simulink model "flightControlSystem"  (R2022a)
settings: Solver=ode3  StartTime=0  StopTime=TFinal  FixedStep=Ts  RelTol=1e-3  EnableMultiTasking=on
model workspace (MAT data in the model file):
  CIRCLE_PTS = [19 19 19]
  ZEROS = [0 0 0 0 0 0 0 0 0 0 0 0 ... (1444 elements, 38x38)]
undefined symbols (not defined in the file): codertarget, Controller, DiscIntNeverNeededParam, Discrete, Estimator, g, gray, init, Sensors, Time, Ts, var_acc_angle_N, var_bias_gyr_N, var_gyro_p_N, Vehicle
libraries: simulink x38, slpidlib x4, ctrlSharedLib x4, sharedtransform x3, visiontextngfix x1, parrotlib x1
(part 3 of 3)

== matlab function flightControlSystem/Image Processing System/write_or_not ==
  data: way input; way_out output; in_red input; prev_xy input; way_x output; way_y output
function [way_out, way_x, way_y] = fcn(way, in_red, prev_xy)

x = way(1);
y = way(2);
speed = way(3);

if in_red
    X = x;   Y = y;
    way_x = x;  way_y = y;
else
    X = x;  Y = y; 
    way_x = prev_xy(1);  
    way_y = prev_xy(2);
end

way_out = [X Y speed];

%fprintf('X = %f | Y = %f\n', way_x, way_y);
end

== matlab function flightControlSystem/Control System/Controller/Position Controller/Position error transformation (Earth to Body frame) ==
  data: yaw input; xy_err_earth input; xy_err_body output
function xy_err_body = fcn(yaw,xy_err_earth)

transformation = [cos(yaw), sin(yaw); -sin(yaw),  cos(yaw)];
xy_err_body = transformation * xy_err_earth;


end

== matlab function flightControlSystem/Image Processing System/speed_calculator ==
  data: way input; X output; Y output
function [X,Y] = fcn(way)

x = way(1);
y = way(2);
speed = way(3);

if speed == 100
    speed = 200;
elseif speed < 60
    speed = 60;
end


X = (60-x) / 10000000 * speed;
Y = (y-80) / 10000000 * speed;


%fprintf(' --- speed: %f | ', speed); fprintf('vectors: X=%.5f | Y=%.5f\n', X, Y);

end

== matlab function flightControlSystem/Image Processing System/opposite_way ==
  data: way_x output; prev_xy input; way_y output
function [way_x, way_y] = fcn(prev_xy)

    x = prev_xy(1);
    y = prev_xy(2);
    
    if x == 0 || y == 0
        way_x = 0;
        way_y = 0;
    else
        way_x = 60 + (60 - x) + 1;
        way_y = 80 + (80 - y) + 1;
    end

    %fprintf('opposite: %.0f %.0f -> %.0f %.0f\n', x, y, way_x, way_y);
end

== matlab function flightControlSystem/Image Processing System/center_vector_x ==
  data: u input; slide_x output
function slide_x = fcn(u)
c1 = 60; 
c2 = 80;
left_p = 0;
right_p = 0;
middle_point = u(c1, c2);
compare = ~middle_point;
for i = c2:-1:60 % <---  look left
    if u(c1, i) == compare
        left_p = i;
        break
    end
end
for i = c2:100 % --->   look right
    if u(c1, i) == compare
        right_p = i;
        break
    end
end

slide_x = 0;
if left_p ~= 0 && right_p ~= 0 % in line
    if middle_point == 1
        vr = right_p - c2;  % length right 
        vl = c2 - left_p;   % length left
        diff = vr-vl;
        slide_x = get_speed(diff) * 20;
    end
end
end

function T = get_speed(t)

if t > 0
    if t < 1
        T = 0.000001;
    elseif t < 5
        T = 0.000002;
    elseif t < 10
        T = 0.000003;
    elseif t < 15
        T = 0.000004;
    elseif t < 20
        T = 0.000005;
    else
        T = 0.000006;
    end
else
    if t < -20
        T = -0.000006;
    elseif t < -15
        T = -0.000005;
    elseif t < -10
        T = -0.000004;
    elseif t < -5
        T = -0.000003;
    elseif t < -1
        T = -0.000002;
    else
        T = -0.000001;
    end
end

end

== matlab function flightControlSystem/Image Processing System/range_points ==
  data: x input; x1 output; y input; ref input; y1 output; x2 output; y2 output
function [x1,y1, x2,y2] = get_range_points(x,y, ref)

% x1, y1 are left
% x2, y2 are right 
% according to center-to-edge vector.

W = edge_number(x,y);

if W == 1
    y1 = y - ref;
    if y1 < 1
        x1 = x - y1;
        y1 = 1;
    else
        x1 = x;
    end

    y2 = y + ref;
    if y2 > 160
        x2 = y2-160;
        y2 = 160;
    else
        x2 = x;
    end
elseif W == 2
    x1 = x + ref;
    if x1 > 120
        y1 = x1 - 120;
        x1 = 120;
    else
        y1 = y;
    end

    x2 = x - ref;
    if x2 < 1
        y2 = abs(x2) + 1;
        x2 = 1;
    else
        y2 = y;
    end
elseif W == 4
    x1 = x - ref;
    if x1 < 1
        y1 = 160 + x1;
        x1 = 1;
    else
        y1 = 160;
    end

    x2 = x + ref;
    if x2 > 120
        y2 = 160 - (x2 - 120);
        x2 = 120;
    else
        y2 = y;
    end
elseif W == 3
    y1 = y + ref;
    if y1 > 160
        x1 = 120 - (y1-160);
        y1 = 160;
    else
        x1 = x;
    end

    y2 = y - ref;
    if y2 < 1
        x2 = 120 + y2;
        y2 = 1;
    else
        x2 = x;
    end
else
    x1 = 1; y1 = 1;
    x2 = 1; y2 = 2;
end

%fprintf('range_points: %.0f-%.0f  to  %.0f-%.0f\n', x1,y1, x2,y2);

end

== stateflow chart flightControlSystem/Control System/Path Planning/Chart ==
  state hover
    xout = 0;
    yout = 0;
    zout = -1.1;
  state go
    xout = xout + xin;
    yout = yout + yin;
    zout = -1.1;
  state land
    zout = zout + 0.002;
    xout = xout;
    yout = yout;
  (default) -> hover
  go -> land : [land == 1]
  hover -> go : [after(2, sec)]
  data: xout output; yout output; zout output; yin input; xin input; land input

== matlab function flightControlSystem/Control System/Path Planning/way_parser ==
  data: x output; u input; y output; land output
function [x, y, land] = fcn(u)

x = u(1);
y = u(2);
land = u(3);

end

== matlab function flightControlSystem/Image Processing System/center_vector_y ==
  data: u input; slide_y output
function slide_y = fcn(u)
c1 = 60; 
c2 = 80;
up_p = 0;
down_p = 0;
middle_point = u(c1,c2);
compare = ~middle_point;
for i = c1:-1:40 % look up
    if u(i, c2) == compare
        up_p = i;
        break
    end
end
for i = c1:80 % look down
    if u(i, c2) == compare
        down_p = i;
        break
    end
end
slide_y = 0;
if up_p ~= 0 && down_p ~= 0  % in line
    if middle_point == 1
        vu = down_p - c1;  %length up
        vd = c1 - up_p;    %length down
        diff = vd-vu;
        
        slide_y = get_speed(diff) * 20;
    end
end

end
function T = get_speed(t)

if t > 0
    if t <= 1
        T = 0.000001;
    elseif t < 5
        T = 0.000002;
    elseif t < 10
        T = 0.000003;
    elseif t < 15
        T = 0.000005;
    elseif t < 20
        T = 0.000005;
    else
        T = 0.000005;
    end
else
    if t < -20
        T = -0.000005;
    elseif t < -15
        T = -0.000005;
    elseif t < -10
        T = -0.000004;
    elseif t <= -5
        T = -0.000003;
    elseif t < -1
        T = -0.000002;
    else
        T = -0.000001;
    end
end
end

== matlab function flightControlSystem/Image Processing System/scan_range ==
  data: way output; u input; x1 input; y1 input; x2 input; y2 input; is_scan input
function way  = scan_range(u, x1,y1, x2,y2, is_scan)

way_x = 1;
way_y = 2;
speed = 0;
in_red_line = u(60, 80);


persistent prev_endless_x;
persistent prev_endless_y;

if is_scan
    if in_red_line == 1  % ------ inside red-line ------
    
        t = 0;
        mx = 0;

        mx_endless_x = [0 0];
        mx_endless_y = [0 0];
        mx_t = [0 0];

        last_endless = false;
        index_of_endless = 0;
        
        w1 = edge_number(x1,y1);
        xi = x1;  yi = y1; k = 1;
        
        if w1 == 1 || w1 == 4
            k = -1;
        end
        
        
        while xi ~= x2 || yi ~= y2
            returned = line_drawer(60, 80, xi, yi, u, 0);

            if returned == 0 % if endless

                if last_endless == false
                    last_endless = true;
                    index_of_endless = index_of_endless + 1;
                end
                if index_of_endless > 2
                    break;
                end
                
                mx_endless_x(index_of_endless) = mx_endless_x(index_of_endless) + xi;
                mx_endless_y(index_of_endless) = mx_endless_y(index_of_endless) + yi;
                mx_t(index_of_endless) = mx_t(index_of_endless) + 1;

            else
                last_endless = false;
                if returned > mx
                    mx = returned;
                    way_x = xi; 
                    way_y = yi;
                    t = 1;
                end
            end

            % İteration
            temp_w = edge_number(xi, yi);
            if temp_w == 1 || temp_w == 3
                yi = yi + k;
            else
                xi = xi + k;
            end
            if xi < 1
                yi = 159; xi = 1; k = -1;
            elseif xi > 120
                xi = 120; yi = 2; k = 1;
            elseif yi < 1
                yi = 1; xi = 2; k = 1;
            elseif yi > 160
                yi = 160; xi = 119; k = -1;
            end
        end % while end


        if index_of_endless == 1 % ---------- 1 endless ------------
            %fprintf('only one endless!\n');
            way_x = mx_endless_x(1);
            way_y = mx_endless_y(1);
            t = mx_t(1);

            way_x = round(way_x/t);
            way_y = round(way_y/t);
            [way_x, way_y] = nearest_edge(way_x, way_y);

            prev_endless_x = 60 + (60 - way_x) + 1;
            prev_endless_y = 80 + (80 - way_y) + 1;

        elseif index_of_endless == 2 % ---------- 2 endless ------------
            
            if isempty(prev_endless_x)
                way_x = mx_endless_x(1);
                way_y = mx_endless_y(1);
                t = mx_t(1);
    
                way_x = round(way_x/t);
                way_y = round(way_y/t);
                [way_x, way_y] = nearest_edge(way_x, way_y);
    
                prev_endless_x = 60 + (60 - way_x) + 1;
                prev_endless_y = 80 + (80 - way_y) + 1;
            else
                mid_calculated = [0 0; 0 0];
                for i = 1:2
                    x = mx_endless_x(i);
                    y = mx_endless_y(i);
                    t = mx_t(i);

                    x = round(x/t);
                    y = round(y/t);
                    
                    [x,y] = nearest_edge(x, y);
                    
                    mid_calculated(i, 1) = x;
                    mid_calculated(i, 2) = y;
                end
                %fprintf('calculated = %.0f %.0f  | %.0f %.0f\n', ...
                %    mid_calculated(1,1), mid_calculated(1,2), ...
                %    mid_calculated(2,1), mid_calculated(2,2));

                diff_x1 = prev_endless_x-mid_calculated(1,1);
                diff_y1 = prev_endless_y-mid_calculated(1,2);
                diff_x2 = prev_endless_x-mid_calculated(2,1);
                diff_y2 = prev_endless_y-mid_calculated(2,2);
                diff1 = sqrt(diff_x1*diff_x1 + diff_y1*diff_y1);
                diff2 = sqrt(diff_x2*diff_x2 + diff_y2*diff_y2);

                if diff1 > diff2
                    way_x = mid_calculated(1,1);
                    way_y = mid_calculated(1,2);
                else
                    way_x = mid_calculated(2,1);
                    way_y = mid_calculated(2,2);
                end
                
                prev_endless_x = 60 + (60 - way_x) + 1;
                prev_endless_y = 80 + (80 - way_y) + 1;
                
            end
        else % ---------- NO endless ------------
            speed = mx;
        end

        

    else % ----------------- outside red line ----------------------
        x1 = 2; y1 = 1;
        x2 = 1; y2 = 1;
        
        ENDLESS = 100;
        mn = ENDLESS;
        w1 = edge_number(x1,y1);
        xi = x1;  yi = y1;  k = 1;
        if w1 == 1 || w1 == 4
            k = -1;
        end
        
        while xi ~= x2 || yi ~= y2
            returned = line_drawer(60, 80, xi, yi, u, 1);
    
            if returned > 0 && returned < mn
                mn = returned;
                way_x = xi;
                way_y = yi;
            end
    
            % İteration
            temp_w = edge_number(xi, yi);
            if temp_w == 1 || temp_w == 3
                yi = yi + k;
            else
                xi = xi + k;
            end
            if xi < 1
                yi = 159; xi = 1; k = -1;
            elseif xi > 120
                xi = 120; yi = 2; k = 1;
            elseif yi < 1
                yi = 1; xi = 2; k = 1;
            elseif yi > 160
                yi = 160; xi = 119; k = -1;
            end
        end % while
        
        speed = 100;
        if mn < 60
            speed = 60;
        end
    end % if redline end

end % is_scan

way = [way_x, way_y, speed];

end % function end
